simulink model "CurrPowerLimCalc"  (R2024a)
settings: Solver=FixedStepDiscrete  StartTime=0.0  StopTime=10000  RelTol=1e-3
model workspace (MAT data in the model file):
  Active_Scenario_Index = 1
  BattTempInit = 25
  Battery.SOC_LUT = [0.01 0.02 0.03 0.04 0.05 0.06 0.07 0.08 0.09 0.1 0.11 0.12 0.13 0.14 0.15 0.16 0.17 0.18 0.19 0.2 0.21 0.22 0.23 0.24 0.25 0.26 0.27 0.28 0.29 0.3 0.31 0.32 0.33 0.34 0.35 0.36 0.37 0.38 0.39 0.4 0.41 0.42 0.43 0.44 0.45 0.46 0.47 0.48 0.49 0.5 0.51 0.52 0.53 0.54 0.55 0.56 0.57 0.58 0.59 0.6 0.61 0.62 0.63 0.64 0.65 0.66 0.67 0.68 0.69 0.7 0.71 0.72 0.73 0.74 0.75 0.76 0.77 0.78 0.79 0.8 0.81 0.82 0.83 0.84 0.85 0.86 0.87 0.88 0.89 0.9 0.91 0.92 0.93 0.94 0.95 0.96 0.97 0.98 0.99 1]
  Battery.Temperature_LUT = [-10 0 25 40]
  Battery.Capacity_LUT = [4.04528301887 4.19622641509 4.8 4.73962264151]
  Battery.Em_LUT = [2.67308083891 2.74411674384 2.80408613071 2.86247711994 2.90851059763 2.94904306488 2.9829846776 3.01467102589 3.04031502638 3.06256828113 3.08180972392 3.09994219643 ... (400 elements, 100x4)]
  Battery.R0_LUT = [0.0569026752707 0.0575506938969 0.0576730924021 0.0575627404981 0.0573787336615 0.0571931123197 0.0568199985482 0.056411926464 0.0561974340667 0.0560805640861 0.0557640899305 0.055275807865 ... (400 elements, 100x4)]
  Battery.R1_LUT = [0.0035 0.0035 0.0035 0.0035 0.0035 0.0035 0.0035 0.0035 0.0035 0.0035 0.0035 0.0035 ... (400 elements, 100x4)]
  Battery.C1_LUT = [5000 5000 5000 5000 5000 5000 5000 5000 5000 5000 5000 5000 ... (400 elements, 100x4)]
  Battery.Mass = 0.047
  Battery.ThermalMass = 44
  Battery.R_bleed = 20
  Battery.h_conv = 5
  Battery.cell_area = 0.0037
  Battery.TempInit = 25
  Battery.SOCInit = 0.75
  Battery.Model = 'panasonic ncr18650bd'
  Battery.DischargeCycle_LUT = [1 5 9 13 17 21 25 29 33 37 41 45 49 53 57 61 65 69 73 77 81 85 89 93 97 101 105 109 113 117 121 125 129 133 137 141 145 149 153 157 161 165 169 173 177 181 185 189 193 197 201 205 209 213 217 221 225 229 233 237 241 245 249 253 257 261 265 269 273 277 281 285 289 293 297 301 305 309 313 317]
  Battery.deltaEm_LUT = [0 -0.363115641304 -0.600096647258 -0.689070000839 -0.76773380251 -0.846397604181 -0.926368385458 -0.992711297521 -1.05704974111 -1.12227693902 -1.19018070587 -1.25808447272 -1.31699459748 -1.35876443799 -1.40168267642 -1.44460091485 -1.48751915327 -1.5304373917 -1.57335563013 -1.62198241593 -1.67232184498 -1.71858340023 -1.76179802551 -1.8050126508 -1.84822727608 -1.8917937136 -1.93575272784 -1.97971174208 -2.02367075632 -2.06762977056 -2.11171979109 -2.15588700406 -2.19980020032 -2.24365853098 -2.28751686164 -2.33137519231 -2.37523352297 -2.41909185363 -2.45982559031 -2.49599372373 -2.53216185715 -2.56832999058 -2.604498124 -2.64066625743 -2.67683439085 -2.71300252428 -2.7491706577 -2.78367585394 -2.81632179346 -2.8483348579 -2.88034792233 -2.91236098677 -2.94437405121 -2.97638711564 -3.00840018008 -3.04041324451 -3.07260346059 -3.10359008254 -3.13082308991 -3.15805609728 -3.18528910464 -3.21252211201 -3.23975511938 -3.26698812675 -3.29422113412 -3.32122400938 -3.3463475604 -3.37152613073 -3.39670470105 -3.42188327138 -3.4470618417 -3.47224041203 -3.49938358795 -3.52900276724 -3.55862194653 -3.58824112582 -3.6178603051 -3.64748858268 -3.67711690909 -3.70674523549]
  Battery.deltaCapacity_LUT = [0 -0.860019120059 -1.71332421702 -2.0819400264 -2.45055583577 -2.81917164515 -3.18778745452 -3.48884924257 -3.7808148236 -4.07278040463 -4.36474598566 -4.6567115667 -4.91000721732 -5.08494410056 -5.2598809838 -5.43481786703 -5.60975475027 -5.78469163351 -5.95962851674 -6.13456539998 -6.30950228322 -6.47026795816 -6.62044510558 -6.77062225299 -6.92079940041 -7.07097654783 -7.22115369524 -7.37133084266 -7.52150799007 -7.67168513749 -7.82230984162 -7.97319825819 -8.12408667477 -8.27497509134 -8.42586350792 -8.57675192449 -8.72764034107 -8.87852875764 -9.01789522921 -9.13717923376 -9.25646323831 -9.37574724285 -9.4950312474 -9.61431525195 -9.73359925649 -9.85288326104 -9.97216726558 -10.0914512701 -10.2059878191 -10.3183039593 -10.4306200996 -10.5429362398 -10.65525238 -10.7675685203 -10.8798846605 -10.9922008008 -11.104516941 -11.2125891929 -11.3075699376 -11.4025506823 -11.4975314271 -11.5925121718 -11.6874929166 -11.7824736613 -11.877454406 -11.9716325175 -12.0588579537 -12.1460833899 -12.2333088261 -12.3205342623 -12.4077596986 -12.4949851348 -12.5890165008 -12.6916254178 -12.7942343349 -12.8968432519 -12.999452169 -13.102061086 -13.2046700031 -13.3072789201]
  Battery.cond_thickness = 0.001
  Battery.thermal_conductivity = 205
  CellType = 1
  HighTempDchrgCurrentLim = Simulink.Signal
  HighTempDchrgCurrentLim.DataType = 'single'
  HighTempDchrgCurrentLim.Dimensions = -1
  HighTempDchrgCurrentLim.DimensionsMode = 'auto'
  HighTempDchrgCurrentLim.Complexity = 'auto'
  HighTempDchrgCurrentLim.SampleTime = -1
  HighTempDchrgCurrentLim.SamplingMode = 'auto'
  LowTempDchrgCurrentLim = Simulink.Signal
  LowTempDchrgCurrentLim.DataType = 'single'
  LowTempDchrgCurrentLim.Dimensions = -1
  LowTempDchrgCurrentLim.DimensionsMode = 'auto'
  LowTempDchrgCurrentLim.Complexity = 'auto'
  LowTempDchrgCurrentLim.SampleTime = -1
  LowTempDchrgCurrentLim.SamplingMode = 'auto'
  MaxChrgCurrLim = Simulink.Parameter
  MaxChrgCurrLim.Value = 6.36000013351
  MaxChrgCurrLim.Complexity = 'real'
  MaxChrgCurrLim.Dimensions = [1 1]
  MaxChrgCurrLim.DataType = 'single'
  MaxDchrgCurrLim = Simulink.Parameter
  MaxDchrgCurrLim.Value = -20
  MaxDchrgCurrLim.Complexity = 'real'
  MaxDchrgCurrLim.Dimensions = [1 1]
  MaxDchrgCurrLim.DataType = 'single'
  MinCellVoltDchrgCurrentLim = Simulink.Signal
  MinCellVoltDchrgCurrentLim.DataType = 'single'
  MinCellVoltDchrgCurrentLim.Dimensions = -1
  MinCellVoltDchrgCurrentLim.DimensionsMode = 'auto'
  MinCellVoltDchrgCurrentLim.Complexity = 'auto'
  MinCellVoltDchrgCurrentLim.SampleTime = -1
  MinCellVoltDchrgCurrentLim.SamplingMode = 'auto'
  MinCellVoltDchrgCurrentLimTable = Simulink.LookupTable
  MinCellVoltDchrgCurrentLimTable.Table = Simulink.lookuptable.Table
  MinCellVoltDchrgCurrentLimTable.Table.Value = [0 0.5 1]
  MinCellVoltDchrgCurrentLimTable.Table.Dimensions = [1 3]
  MinCellVoltDchrgCurrentLimTable.Table.DataType = 'single'
  MinCellVoltDchrgCurrentLimTable.Table.FieldName = 'DischargeCurrentRate'
  MinCellVoltDchrgCurrentLimTable.Table.Description = 'Discharge Current Rate Based On Mim Cell Voltage'
  MinCellVoltDchrgCurrentLimTable.Breakpoints = Simulink.lookuptable.Breakpoint
  MinCellVoltDchrgCurrentLimTable.Breakpoints.Value = [2.5; 2.75; 3]
  MinCellVoltDchrgCurrentLimTable.Breakpoints.TunableSizeName = 'N1'
  MinCellVoltDchrgCurrentLimTable.Breakpoints.Dimensions = [3 1]
  MinCellVoltDchrgCurrentLimTable.Breakpoints.DataType = 'single'
  MinCellVoltDchrgCurrentLimTable.Breakpoints.Unit = 'V'
  MinCellVoltDchrgCurrentLimTable.Breakpoints.FieldName = 'MinCellVoltage'
  MinCellVoltDchrgCurrentLimTable.Breakpoints.Description = 'Minimum Cell Voltage'
  MinCellVoltDchrgCurrentLimTable.AllowMultipleInstancesOfTypeToHaveDifferentTableBreakpointSizes = 0
  MinCellVoltDchrgCurrentLimTable.SupportTunableSize = 0
  MinCellVoltDchrgCurrentLimTable.StructTypeInfo = Simulink.lookuptable.StructTypeInfo
  MinCellVoltDchrgCurrentLimTable.StructTypeInfo.Name = 'MinCellVoltDchrgCurrentLimTable'
  MinCellVoltDchrgCurrentLimTable.StructTypeInfo.DataScope = 'Auto'
  Np_Module = 31
  Ns_Module = 24
  NumModules = 4
  OverCellVoltageLimit = 4.19999980927
  TestCase = 1
  UnderCellVoltageLimit = 2.5
  ts = 0.1
undefined symbols (not defined in the file or in its folder): MinCellVoltDchrgCurrentLim_BP, MinCellVoltDchrgCurrentLim_Table
settings Model: DataDictionary=DD_CurrPowerLimCalc.sldd  ModifiedByFormat=The MathWorks, Inc.  ExtModeTrigDuration=5  Creator=The MathWorks, Inc.  LastModifiedBy=The MathWorks, Inc.
settings SolverCC: AlgebraicLoopSolver=TrustRegion  PositivePriorityOrder=on  AutoInsertRateTranBlk=on  MaxZcPerStep=1
settings DataIOCC: ExternalInput=Battery  SaveOutput=off  SaveTime=off  SignalLoggingName=logsOut
settings OptimizationCC: BlockReduction=off  DefaultParameterBehavior=Inlined  UseFloatMulNetSlope=on  DefaultUnderspecifiedDataType=single  EnhancedBackFolding=on  PassReuseOutputArgsAs=Individual arguments  ZeroExternalMemoryAtStartup=off  ZeroInternalMemoryAtStartup=off  EfficientFloat2IntCast=on  MaxStackSize=64  OptimizeBlockOrder=speed  DifferentSizesBufferReuse=on  OptimizationCustomize=off  EfficientTunableParamExpr=on
settings DebuggingCC: SignalInfNanChecking=error  SaveWithParameterizedLinksMsg=none  CheckExecutionContextPreStartOutputMsg=on  IntegerOverflowMsg=error  ParameterPrecisionLossMsg=none  ParameterTunabilityLossMsg=error  UnconnectedInputMsg=warning  UnconnectedOutputMsg=warning  UnconnectedLineMsg=warning  AssertControl=DisableAll  PregeneratedLibrarySubsystemCodeDiagnostic=none  SubsystemReferenceDiagnosticForUnitTest=warning  SFUnexpectedBacktrackingDiag=warning  SFNoUnconditionalDefaultTransitionDiag=warning  SFExecutionAtInitializationDiag=none  ArithmeticOperatorsInVariantConditions=warning
settings HardwareCC: ProdBitPerLong=64  ProdLongLongMode=on  ProdHWDeviceType=Intel->x86-64 (Linux 64)
settings ModelReferenceCC: EnableRefExpFcnMdlSchedulingChecks=on  ModelReferenceNumInstancesAllowed=Single  PropagateSignalLabelsOutOfModel=off
settings SFSimCC: SimUseLocalCustomCode=off  MATLABDynamicMemAlloc=off  CustomCodeUndefinedFunction=UseInterfaceOnly
settings RTWCC: Description=AUTOSAR  SystemTargetFile=autosar.tlc  GenCodeOnly=on  TemplateMakefile=ert_default_tmf  GenerateReport=on  RTWUseLocalCustomCode=off  Toolchain=Simulink Real-Time Toolchain  BuildConfiguration=Faster Runs  GPUComputeCapability=3.5  DLArmComputeVersion=19.05
settings CodeAppCC: ForceParamTrailComments=on  IgnoreCustomStorageClasses=off  MaxIdLength=51  OperatorAnnotations=on  SimulinkDataObjDesc=on  SFDataObjDesc=on  MangleLength=4  InsertBlockDesc=on
settings STFCustomTargetCC: MultiwordLength=256  ParMdlRefBuildCompliant=on  CompOptLevelCompliant=on  IncludeMdlTerminateFcn=off  CombineOutputUpdateFcns=on  SuppressErrorStatus=on  ERTCustomFileBanners=on  SupportComplex=off  SupportContinuousTime=off  SupportNonInlinedSFcns=off  RemoveResetFunc=on  SupportVariableSizeSignals=on  MATLABClassNameForMDSCustomization=Simulink.SoftwareTarget.ERTCustomization  AutosarCompliant=on  GRTInterface=off  LookupTableObjectStructAxisOrder=2,1,3,4,...  LUTObjectStructOrderEvenSpacing=Size,Table,Breakpoints  SystemTargetFile=autosar.tlc
settings ERTTargetCC: TargetLangStandard=C99 (ISO)  ConcurrentExecutionCompliant=off  IncludeMdlTerminateFcn=off  SuppressErrorStatus=on  SupportComplex=off  SupportVariableSizeSignals=on  ModelStepFunctionPrototypeControlCompliant=off  CPPClassGenCompliant=off  AutosarCompliant=on  LookupTableObjectStructAxisOrder=2,1,3,4,...  LUTObjectStructOrderEvenSpacing=Size,Table,Breakpoints  InlinedParameterPlacement=NonHierarchical  ERTCustomFileTemplate=example_file_process.tlc
settings ConfigComp: CovMetricSettings=dcw  CovSaveCumulativeToWorkspaceVar=on  CovSaveSingleToWorkspaceVar=on  CovExternalEMLEnable=off  CovSFcnEnable=off  DVMode=DesignErrorDetection  DVMaxProcessTime=7000  DVTestSuiteOptimization=Auto  DVDetectDeadLogic=on  DVDetectIntegerOverflow=off  DVRebuildModelRepresentation=Always

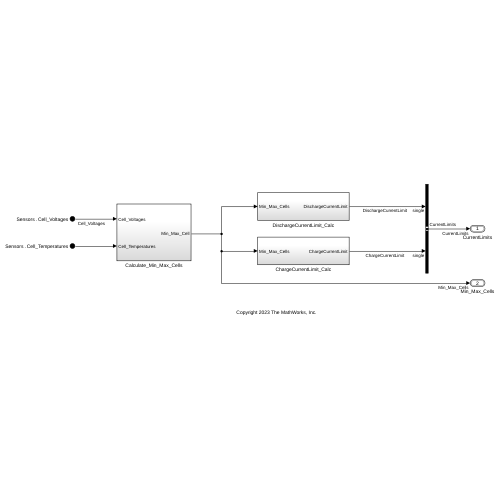
[thumbnail: Simulink's stored preview of the top-level diagram]
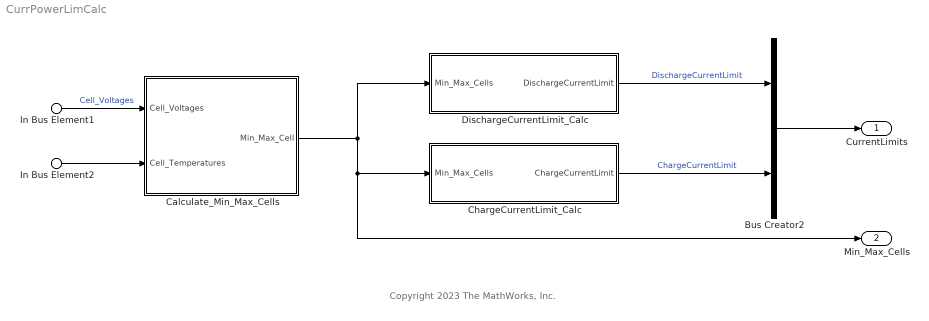
== system CurrPowerLimCalc ==
  note: Copyright 2023 The MathWorks, Inc.
  In Bus Element1 : Inport  PortName=Sensors  Element=Cell_Voltages
  In Bus Element2 : Inport  PortName=Sensors  Element=Cell_Temperatures
  Bus Creator2 : BusCreator  Inputs=2  OutDataTypeStr=Bus: CurrentLimits  NonVirtualBus=on
  Calculate_Min_Max_Cells : Subsystem
  ChargeCurrentLimit_Calc : Subsystem
  DischargeCurrentLimit_Calc : Subsystem
  CurrentLimits : Outport  OutDataTypeStr=Bus: CurrentLimits  BusOutputAsStruct=on
  Min_Max_Cells : Outport  Port=2  OutDataTypeStr=Bus: Min_Max_Cells  BusOutputAsStruct=on
  wires:
  In Bus Element1/1 -> Calculate_Min_Max_Cells/1(Cell_Voltages)  "Cell_Voltages"
  In Bus Element2/1 -> Calculate_Min_Max_Cells/2(Cell_Temperatures)
  Bus Creator2/1 -> CurrentLimits/1
  ChargeCurrentLimit_Calc/1(ChargeCurrentLimit) -> Bus Creator2/2  "ChargeCurrentLimit"
  DischargeCurrentLimit_Calc/1(DischargeCurrentLimit) -> Bus Creator2/1  "DischargeCurrentLimit"
  Calculate_Min_Max_Cells/1(Min_Max_Cell) -> Min_Max_Cells/1, ChargeCurrentLimit_Calc/1(Min_Max_Cells), DischargeCurrentLimit_Calc/1(Min_Max_Cells)

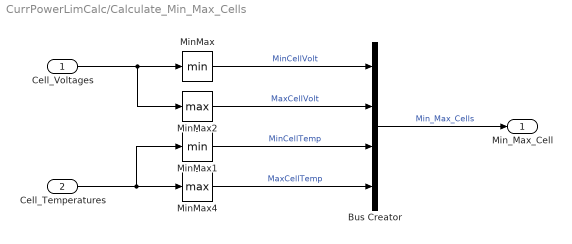
== system CurrPowerLimCalc/Calculate_Min_Max_Cells ==
  Cell_Voltages : Inport
  Cell_Temperatures : Inport  Port=2
  Bus Creator : BusCreator  Inputs=4  OutDataTypeStr=Bus: Min_Max_Cells  NonVirtualBus=on
      settings: InheritFromInputs=off
  MinMax : MinMax
  MinMax1 : MinMax
  MinMax2 : MinMax  Function=max
  MinMax4 : MinMax  Function=max
  Min_Max_Cell : Outport  OutDataTypeStr=Bus: Min_Max_Cells  PortDimensions=1  SampleTime=[0.10000000000000001,0]  VectorParamsAs1DForOutWhenUnconnected=off
  wires:
  MinMax2/1 -> Bus Creator/2  "MaxCellVolt"
  Cell_Temperatures/1 -> MinMax4/1, MinMax1/1
  MinMax/1 -> Bus Creator/1  "MinCellVolt"
  Cell_Voltages/1 -> MinMax/1, MinMax2/1
  MinMax1/1 -> Bus Creator/3  "MinCellTemp"
  MinMax4/1 -> Bus Creator/4  "MaxCellTemp"
  Bus Creator/1 -> Min_Max_Cell/1  "Min_Max_Cells"

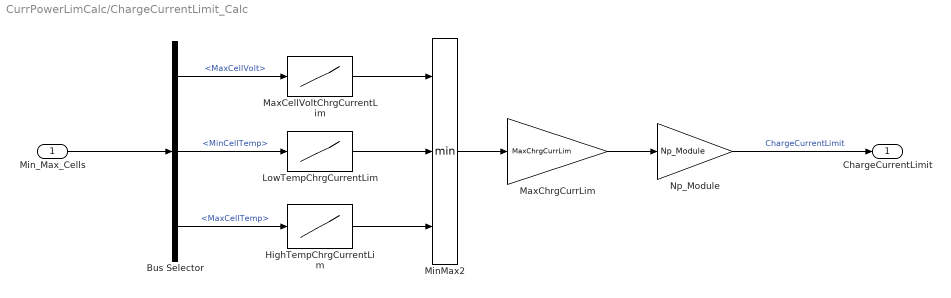
== system CurrPowerLimCalc/ChargeCurrentLimit_Calc ==
  Min_Max_Cells : Inport
  Bus Selector : BusSelector  OutputSignals=MaxCellVolt,MinCellTemp,MaxCellTemp
  HighTempChrgCurrentLim : Lookup_n-D  NumberOfTableDimensions=1  BreakpointsForDimension1="single([40  45  50  55 60])"  Table=single([1.0 0.8 0.5 0.3 0])  ExtrapMethod=Clip  InternalRulePriority=Speed  RndMeth=Simplest
  LowTempChrgCurrentLim : Lookup_n-D  NumberOfTableDimensions=1  BreakpointsForDimension1=single([-15 -10 -5.0 0.0 5.0 10 15.0])  Table="single([0.1 0.2  0.3 0.3 0.5 1.0 1.0])"  ExtrapMethod=Clip  InternalRulePriority=Speed  RndMeth=Simplest
  MaxCellVoltChrgCurrentLim : Lookup_n-D  NumberOfTableDimensions=1  BreakpointsForDimension1=single([3.9 4.0 4.15 4.2])  Table="single([1.0 0.8 0.3  0.3])"  ExtrapMethod=Clip  InternalRulePriority=Speed  RndMeth=Simplest
  MaxChrgCurrLim : Gain  Gain=MaxChrgCurrLim
  MinMax2 : MinMax  Inputs=3
  Np_Module : Gain  Gain=Np_Module
  ChargeCurrentLimit : Outport  VectorParamsAs1DForOutWhenUnconnected=off
  wires:
  MinMax2/1 -> MaxChrgCurrLim/1
  HighTempChrgCurrentLim/1 -> MinMax2/3
  LowTempChrgCurrentLim/1 -> MinMax2/2
  MaxChrgCurrLim/1 -> Np_Module/1
  Min_Max_Cells/1 -> Bus Selector/1
  Bus Selector/2 -> LowTempChrgCurrentLim/1  "<MinCellTemp>"
  Bus Selector/3 -> HighTempChrgCurrentLim/1  "<MaxCellTemp>"
  MaxCellVoltChrgCurrentLim/1 -> MinMax2/1
  Bus Selector/1 -> MaxCellVoltChrgCurrentLim/1  "<MaxCellVolt>"
  Np_Module/1 -> ChargeCurrentLimit/1  "ChargeCurrentLimit"

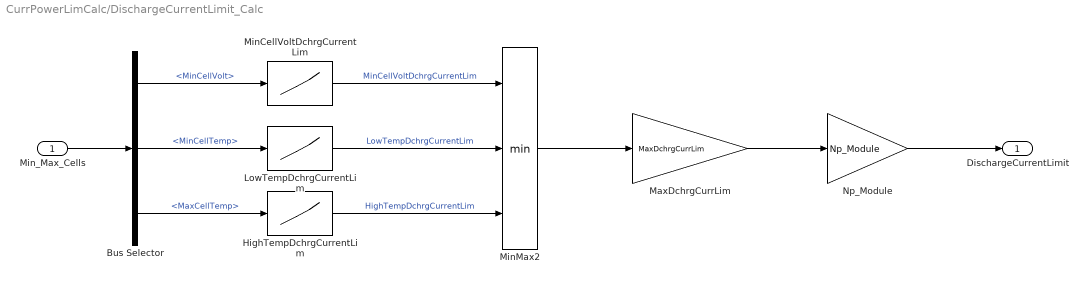
== system CurrPowerLimCalc/DischargeCurrentLimit_Calc ==
  Min_Max_Cells : Inport
  Bus Selector : BusSelector  OutputSignals=MinCellVolt,MinCellTemp,MaxCellTemp
  HighTempDchrgCurrentLim : Lookup_n-D  NumberOfTableDimensions=1  BreakpointsForDimension1=single([40, 45, 50, 60])  Table=single([1, 0.5, 0.3, 0])  ExtrapMethod=Clip  InternalRulePriority=Speed  RndMeth=Simplest
  LowTempDchrgCurrentLim : Lookup_n-D  NumberOfTableDimensions=1  BreakpointsForDimension1="single([-10, -5,    0,   5, 10, 15, 20])"  Table="single([0,  0.2, 0.3, 0.5, 0.75, 1, 1])"  ExtrapMethod=Clip  InternalRulePriority=Speed  RndMeth=Simplest
  MaxDchrgCurrLim : Gain  Gain=MaxDchrgCurrLim
  MinCellVoltDchrgCurrentLim : Lookup_n-D  NumberOfTableDimensions=1  DataSpecification=Lookup table object  LookupTableObject=MinCellVoltDchrgCurrentLimTable  BreakpointsForDimension1=MinCellVoltDchrgCurrentLim_BP  Table=MinCellVoltDchrgCurrentLim_Table  ExtrapMethod=Clip  InternalRulePriority=Speed  RndMeth=Simplest
  MinMax2 : MinMax  Inputs=3
  Np_Module : Gain  Gain=Np_Module
  DischargeCurrentLimit : Outport  VectorParamsAs1DForOutWhenUnconnected=off
  wires:
  MinMax2/1 -> MaxDchrgCurrLim/1
  MaxDchrgCurrLim/1 -> Np_Module/1
  Bus Selector/3 -> HighTempDchrgCurrentLim/1  "<MaxCellTemp>"
  Bus Selector/2 -> LowTempDchrgCurrentLim/1  "<MinCellTemp>"
  HighTempDchrgCurrentLim/1 -> MinMax2/3  "HighTempDchrgCurrentLim"
  LowTempDchrgCurrentLim/1 -> MinMax2/2  "LowTempDchrgCurrentLim"
  Np_Module/1 -> DischargeCurrentLimit/1
  Min_Max_Cells/1 -> Bus Selector/1
  MinCellVoltDchrgCurrentLim/1 -> MinMax2/1  "MinCellVoltDchrgCurrentLim"
  Bus Selector/1 -> MinCellVoltDchrgCurrentLim/1  "<MinCellVolt>"
